simulink model "Lyp2"  (R2018b)
settings: Solver=FixedStepAuto  StartTime=0.0  StopTime=100  FixedStep=0.001  RelTol=1e-3  EnableMultiTasking=on
InitFcn:
  | X0 = randn(1)*10 ;
settings Model: Creator=omid_zandi  LastModifiedBy=Arash
settings OptimizationCC: LifeSpan=inf
settings DebuggingCC: SFUnexpectedBacktrackingDiag=warning  SFNoUnconditionalDefaultTransitionDiag=warning
settings SFSimCC: SimUseLocalCustomCode=off
settings RTWCC: RTWUseLocalCustomCode=off
settings CodeAppCC: StateflowObjectComments=on
settings GRTTargetCC: TargetLangStandard=C89/C90 (ANSI)  GeneratePreprocessorConditionals=Disable all
settings ConfigComp: CovMetricSettings=dw  CovHtmlReporting=on  CovSaveCumulativeToWorkspaceVar=on  CovSaveSingleToWorkspaceVar=on  CovExternalEMLEnable=off

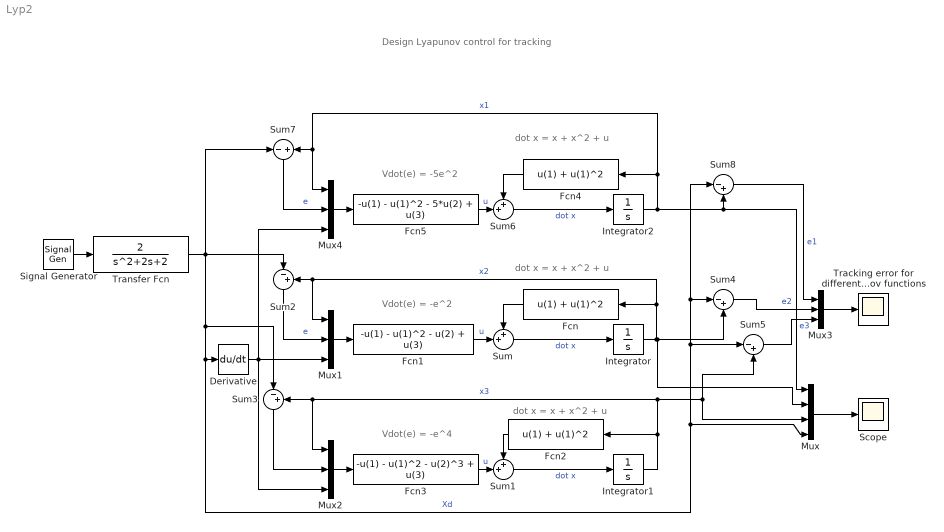
== system Lyp2 ==
  note: Vdot(e) = -e^4
  note: Vdot(e) = -e^2
  note: Design Lyapunov control for tracking
  note: dot x = x + x^2 + u
  note: dot x = x + x^2 + u
  note: Vdot(e) = -5e^2
  note: dot x = x + x^2 + u
  Derivative : Derivative
  Fcn : Fcn  Expr=u(1) + u(1)^2
  Fcn1 : Fcn  Expr=-u(1) - u(1)^2 - u(2) + u(3)
  Fcn2 : Fcn  Expr=u(1) + u(1)^2
  Fcn3 : Fcn  Expr=-u(1) - u(1)^2 - u(2)^3 + u(3)
  Fcn4 : Fcn  Expr=u(1) + u(1)^2
  Fcn5 : Fcn  Expr=-u(1) - u(1)^2 - 5*u(2) + u(3)
  Integrator : Integrator  InitialCondition=X0
  Integrator1 : Integrator  InitialCondition=X0
  Integrator2 : Integrator  InitialCondition=X0
  Mux : Mux
  Mux{1..4} (4 alike) : Mux  Inputs=3
  Scope : Scope
  Signal Generator : SignalGenerator  Frequency=0.05
  Sum : Sum  Inputs=++|
  Sum1 : Sum  Inputs=++|
  Sum{2..5,8} (5 alike) : Sum  Inputs=|-+
  Sum6 : Sum  Inputs=++|
  Sum7 : Sum  Inputs=-|+
  Tracking error for different lyapunov functions : Scope
  Transfer Fcn : TransferFcn  Numerator=[2]  Denominator=[1 2 2 ]
  wires:
  Integrator/1 -> Mux/2, Sum4/2, Mux1/1, Sum2/2, Fcn/1  "x2"
  Sum/1 -> Integrator/1  "dot x"
  Fcn/1 -> Sum/1
  Fcn1/1 -> Sum/2  "u"
  Integrator1/1 -> Mux/3, Sum5/2, Sum3/2, Mux2/1, Fcn2/1  "x3"
  Sum1/1 -> Integrator1/1  "dot x"
  Fcn2/1 -> Sum1/1
  Fcn3/1 -> Sum1/2  "u"
  Mux/1 -> Scope/1
  Signal Generator/1 -> Transfer Fcn/1
  Sum2/1 -> Mux1/2  "e"
  Mux1/1 -> Fcn1/1
  Mux2/1 -> Fcn3/1
  Sum3/1 -> Mux2/2
  Sum4/1 -> Mux3/2  "e2"
  Sum5/1 -> Mux3/3  "e3"
  Mux3/1 -> Tracking error for different lyapunov functions/1
  Sum7/1 -> Mux4/2  "e"
  Transfer Fcn/1 -> Sum2/1, Sum7/1, Sum3/1, Mux/4, Sum5/1, Sum8/1, Sum4/1, Derivative/1  "Xd"
  Mux4/1 -> Fcn5/1
  Integrator2/1 -> Mux/1, Sum8/2, Fcn4/1, Mux4/1, Sum7/2  "x1"
  Fcn5/1 -> Sum6/2  "u"
  Derivative/1 -> Mux4/3, Mux2/3, Mux1/3
  Sum6/1 -> Integrator2/1  "dot x"
  Fcn4/1 -> Sum6/1
  Sum8/1 -> Mux3/1  "e1"
